simulink model "simTwoTag"  (R2023b)
settings: Solver=VariableStepAuto  StartTime=0.0  StopTime=10.0  RelTol=1e-3
undefined symbols (not defined in the file or in its folder): designMultirateFIR, get, hot, magnitude, paramWidebandRadar
libraries: phasedenvlib x4, phaseddetectlib x3, phasedtxrxlib x2, radarlib x2, simulink x1, phasedwavlib x1, dspobslib x1, dspmlti4 x1, dspsigops x1, dspmathops x1, phasedmisclib x1
settings Model: Creator=ericdvet  LastModifiedBy=ericdvet

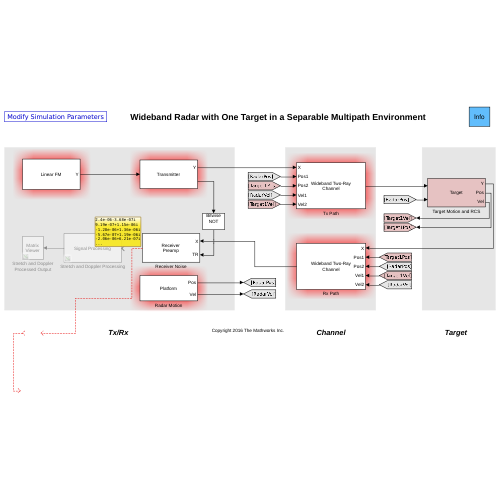
[thumbnail: Simulink's stored preview of the top-level diagram]
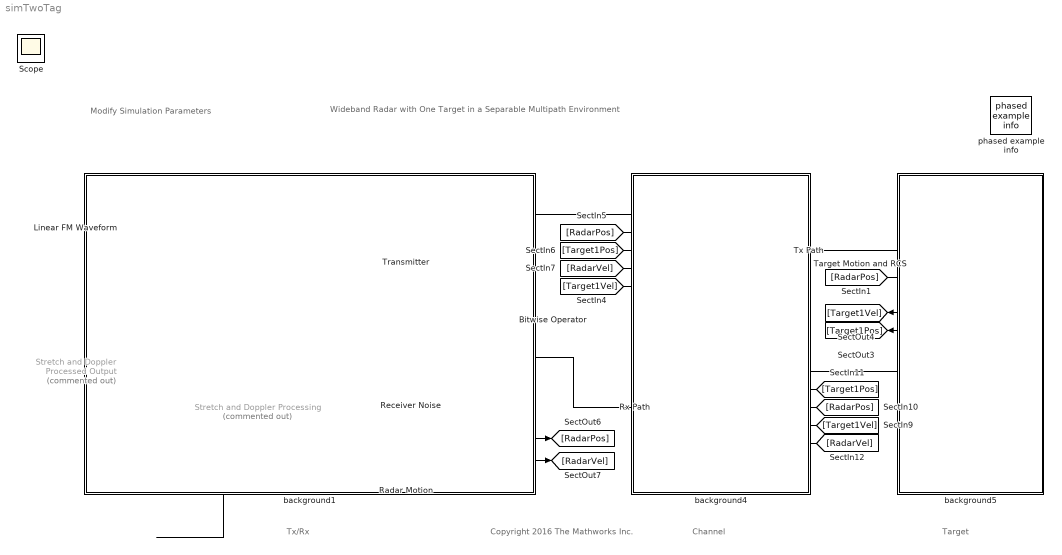
== system simTwoTag ==
  note: Wideband Radar with One Target in a Separable Multipath Environment
  note: Target
  note: Tx/Rx
  note: Copyright 2016 The Mathworks Inc.
  note: Modify Simulation Parameters
  note: Channel
  Bitwise Operator : simulink/Logic and Bit Operations/Bitwise Operator  logicop=NOT  UseBitMask=off  BitMask=bin2dec('11011001')  BitMaskRealWorld=Stored Integer
  Linear FM Waveform : phasedwavlib/Linear FM Waveform  SampleRate=paramWidebandRadar.fs  DurationSpecification=Pulse width  PulseWidth=paramWidebandRadar.pulseWidth  DutyCycle=0.5  PRF=paramWidebandRadar.prf  PRFSelectionInputPort=off  SimulationTimeSource=Derive from waveform parameters  SweepBandwidth=paramWidebandRadar.pulseBw  SweepDirection=Up  SweepInterval=Positive  Envelope=Rectangular  FrequencyOffsetSource=Property  FrequencyOffset=0  OutputFormat=Pulses  NumSamples=100  NumPulses=1  PRFOutputPort=off  CoefficientsOutputPort=off  SimulateUsing=Interpreted execution
  Radar Motion : phasedenvlib/Motion Platform  MotionModel=Velocity  InitialPosition=paramWidebandRadar.sensorPos  InitialVelocity=[ 0; 0; 0 ]  VelocitySource=Property  Velocity=paramWidebandRadar.sensorVel  AccelerationSource=Property  Acceleration=[0;0;0]  CustomTrajectory=[ 0, 0, 0, 0, 0, 0, 0; 1, 0, 0, 0, 0, 0, 0 ]  ScanMode=None  InitialScanAngle=0  AzimuthSpan=[ -60, 60 ]  AzimuthScanRate=10  InitialOrientationAxes=eye( 3 )  OrientationAxesOutputPort=off  ElapsedTimeSource=Auto  SampleRateFromInputCheckbox=on  SampleRate=1e6  SimulateUsing=Interpreted execution
  Receiver Noise : phasedtxrxlib/Receiver Preamp  Gain=20  LossFactor=0  NoiseMethod=Noise temperature  NoiseFigure=0  ReferenceTemperature=290  SampleRateFromInputCheckbox=on  SampleRate=1e6  NoisePower=0  EnableInputPort=on  PhaseNoiseInputPort=off  SeedSource=Auto  Seed=0  SimulateUsing=Interpreted execution
  Rx Path : radarlib/Wideband Two-Ray Channel  PropagationSpeed=paramWidebandRadar.propSpeed  OperatingFrequency=paramWidebandRadar.fc  NumSubbands=paramWidebandRadar.numSubbands  SpecifyAtmosphere=off  Temperature=15  DryAirPressure=101325  WaterVapourDensity=7.5  LiquidWaterDensity=0  RainRate=0  SampleRateFromInputCheckbox=on  SampleRate=1e6  GroundReflectionCoefficient=paramWidebandRadar.groundCoefficient  GroundRelativePermittivity=15  CombinedRaysOutput=on  MaximumDistanceSource=Property  MaximumDistance=10e3  MaximumNumInputSamplesSource=Auto  MaximumNumInputSamples=1000  SimulateUsing=Interpreted execution
  Stretch and Doppler Processed Output : dspobslib/Matrix Viewer  Commented=on  ImageParams=off  CMapStr=hot(256)  AxisColorbar=on  AxisParams=off  AxisOrigin=Lower left corner  AxisTickMode=User-defined  XTickRange=paramWidebandRadar.radialSpeedLim  YTickRange=paramWidebandRadar.rangeLim  XLabel=Radial Speed (m/s)  YLabel=Range (m)  ZLabel=SINR (dB)  FigPos=get(0,'defaultfigureposition')  AxisZoom=off
      settings: YMin=5  YMax=20
  Stretch and Doppler Processing : Subsystem  Commented=on
      mask Display: disp('Signal Processing')
  Target Motion and RCS : Subsystem
      mask Display:
      | disp('Target')
      | port_label('output',1,'Y');
      | port_label('output',2,'Pos');
      | port_label('output',3,'Vel');
  Transmitter : phasedtxrxlib/Transmitter  PeakPower=paramWidebandRadar.peakPower  Gain=paramWidebandRadar.txGain  LossFactor=0  InUseOutputPort=on  CoherentOnTransmit=on  PhaseNoiseOutputPort=off  SeedSource=Auto  Seed=0  SimulateUsing=Interpreted execution
  Tx Path : radarlib/Wideband Two-Ray Channel  PropagationSpeed=paramWidebandRadar.propSpeed  OperatingFrequency=paramWidebandRadar.fc  NumSubbands=paramWidebandRadar.numSubbands  SpecifyAtmosphere=off  Temperature=15  DryAirPressure=101325  WaterVapourDensity=7.5  LiquidWaterDensity=0  RainRate=0  SampleRateFromInputCheckbox=on  SampleRate=1e6  GroundReflectionCoefficient=paramWidebandRadar.groundCoefficient  GroundRelativePermittivity=15  CombinedRaysOutput=on  MaximumDistanceSource=Property  MaximumDistance=10e3  MaximumNumInputSamplesSource=Auto  MaximumNumInputSamples=1000  SimulateUsing=Interpreted execution
  background1 : Subsystem  Description=Jammer
      mask Display: disp('')
  background4 : Subsystem  Description=Jammer
      mask Display: disp('')
  background5 : Subsystem  Description=Jammer
      mask Display: disp('')
  phased example info : phasedmisclib/phased example info  SystemSampleTime=-1  VariantActivationTime=update diagram  AllowFlexibleInterface=on  Latency=0  AutoFrameSizeCalculation=off
  Scope : Scope
  wires:
  Bitwise Operator/1 -> Receiver Noise/2
  Radar Motion/2 -> [RadarVel]
  [Target1Pos] -> Tx Path/3
  Transmitter/2 -> Bitwise Operator/1
  Linear FM Waveform/1 -> Transmitter/1
  [Target1Pos] -> Rx Path/2
  Target Motion and RCS/2(Target Position) -> [Target1Pos]
  Target Motion and RCS/3(Target Velocity) -> [Target1Vel]
  [RadarPos] -> Tx Path/2
  Radar Motion/1 -> [RadarPos]
  Stretch and Doppler Processing/1(Out2) -> Stretch and Doppler Processed Output/1
  [RadarVel] -> Tx Path/4
  [RadarPos] -> Target Motion and RCS/2(In2)
  [Target1Vel] -> Tx Path/5
  [RadarPos] -> Rx Path/3
  Tx Path/1 -> Target Motion and RCS/1(In1)
  Target Motion and RCS/1(Out1) -> Rx Path/1
  [RadarVel] -> Rx Path/5
  [Target1Vel] -> Rx Path/4
  Transmitter/1 -> Tx Path/1
  Rx Path/1 -> Receiver Noise/1
  Receiver Noise/1 -> ?
  ? -> ?

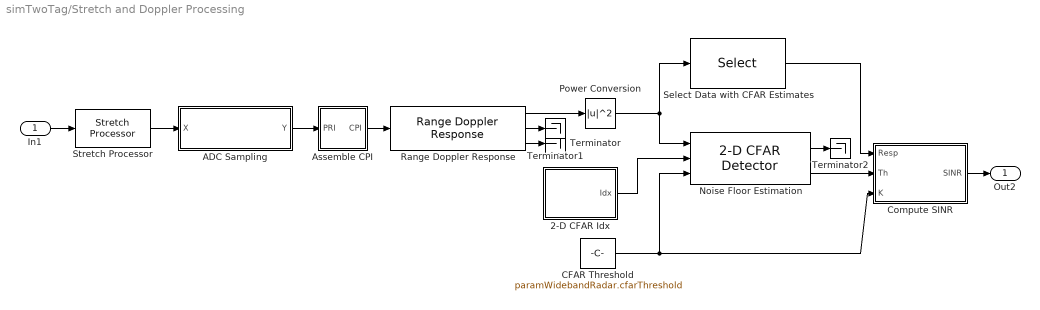
== system simTwoTag/Stretch and Doppler Processing ==
  In1 : Inport
  2-D CFAR Idx : MATLAB Function  TreatAsAtomicUnit=on  mask(2-D CFAR CUT Region){iCUTRng=paramWidebandRadar.cfarRngIdx(1):paramWidebandRadar.cfarRngIdx(2), iCUTDop=paramWidebandRadar.cfarSpdIdx(1):paramWidebandRadar.cfarSpdIdx(2)}
      mask prompts: iCUTRng "Range cells under test:"; iCUTDop "Doppler cells under test:"
      mask help: Generates 2-D CFAR CUT indicies to cover the 2-D region defined by the cell under test (CUT) indicies specified for both range and Doppler.
  ADC Sampling : Subsystem  mask(Decimator){M=paramWidebandRadar.decimateFactor}
      mask prompts: M "Decimation factor:"
      mask help: Decimates the sample rate of the received pulse repetition interval (PRI). The input is a column vector representing a full PRI. The output is a column vector representing the PRI sampled at a reduced rate. The reduction in the sampling rate is specified by the decimation factor, M.
      mask Display:
      | fprintf('Decimator');
      | port_label('input',1,'x[n]');
      | port_label('output',1,sprintf('x[%in]',M));
  Assemble CPI : Subsystem  mask(CPI Buffer){N=paramWidebandRadar.numPulseInt}
      mask prompts: N "PRIs per CPI"
      mask help: Buffers N pulse repetition intervals (PRIs) to form a coherent processing interval (CPI) to be used for Doppler processing. The input is a column vector representing a full PRI. The output is a 2-D column vector with each column corresponding to a buffered PRI.
      mask Display: fprintf('%i PRIs',N);
  CFAR Threshold : Constant  Value=paramWidebandRadar.cfarThreshold
  Compute SINR : Subsystem
  Noise Floor Estimation : phaseddetectlib/2-D CFAR Detector  Method=CA  Rank=paramWidebandRadar.cfarRank  GuardBandSize=paramWidebandRadar.numCFARGuard  TrainingBandSize=paramWidebandRadar.numCFARTrain  ThresholdFactor=Input port  ProbabilityFalseAlarm=0.1  CustomThresholdFactor=1  OutputFormat=CUT result  ThresholdOutputPort=on  NoisePowerOutputPort=off  NumDetectionsSource=Auto  NumDetections=1  SimulateUsing=Interpreted execution
  Power Conversion : Math  Operator=magnitude^2  SignedPower=on
  Range Doppler Response : phaseddetectlib/Range Doppler Response  RangeMethod=FFT  PropagationSpeed=paramWidebandRadar.propSpeed  SampleRateFromInputCheckbox=off  SampleRate=paramWidebandRadar.stretchFs  SweepSlope=paramWidebandRadar.stretchSlope  DechirpInput=off  RangeFFTLengthSource=Auto  RangeFFTLength=1024  RangeWindow=Taylor  RangeSidelobeAttenuation=30  CustomRangeWindow=@hamming  ReferenceRangeCentered=on  ReferenceRange=0  MaximumNumInputSamplesSource=Auto  MaximumNumInputSamples=100  PRFSource=Auto  PRF=10e3  DopplerFFTLengthSource=Property  DopplerFFTLength=paramWidebandRadar.numDopBins  DopplerWindow=Taylor  DopplerSidelobeAttenuation=30  CustomDopplerWindow=@hamming  DopplerOutput=Speed  OperatingFrequency=paramWidebandRadar.fc  SimulateUsing=Interpreted execution
  Select Data with CFAR Estimates : Selector  NumberOfDimensions=2  InputPortWidth=3  IndexOptions=Starting index (dialog),Starting index (dialog)  Indices=min(paramWidebandRadar.cfarRngIdx),min(paramWidebandRadar.cfarSpdIdx)  OutputSizes=max(paramWidebandRadar.cfarRngIdx)-min(paramWidebandRadar.cfarRngIdx)+1,max(paramWidebandRadar.cfarSpdIdx)-min(paramWidebandRadar.cfarSpdIdx)+1
  Stretch Processor : phaseddetectlib/Stretch Processor  PulseWidth=paramWidebandRadar.pulseWidth  PRFSource=Property  PRF=paramWidebandRadar.prf  SweepSlope=paramWidebandRadar.stretchSlope  SweepInterval=Positive  PropagationSpeed=paramWidebandRadar.propSpeed  ReferenceRange=paramWidebandRadar.stretchRef  RangeSpan=paramWidebandRadar.stretchSpan  SimulateUsing=Interpreted execution
  Terminator : Terminator
  Terminator1 : Terminator
  Terminator2 : Terminator
  Out2 : Outport
  wires:
  In1/1 -> Stretch Processor/1
  Assemble CPI/1(CPI) -> Range Doppler Response/1
  CFAR Threshold/1 -> Compute SINR/3(K), Noise Floor Estimation/3
  Noise Floor Estimation/1 -> Terminator2/1
  Range Doppler Response/3 -> Terminator/1
  Range Doppler Response/2 -> Terminator1/1
  Range Doppler Response/1 -> Power Conversion/1
  Select Data with CFAR Estimates/1 -> Compute SINR/1(Resp)
  Noise Floor Estimation/2 -> Compute SINR/2(Th)
  Compute SINR/1(SINR) -> Out2/1
  Power Conversion/1 -> Select Data with CFAR Estimates/1, Noise Floor Estimation/1
  Stretch Processor/1 -> ADC Sampling/1(X)
  ADC Sampling/1(Y) -> Assemble CPI/1(PRI)
  2-D CFAR Idx/1(Idx) -> Noise Floor Estimation/2

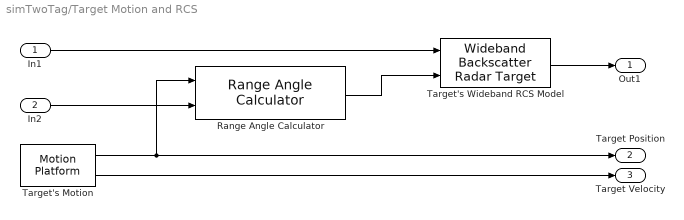
== system simTwoTag/Target Motion and RCS ==
  In1 : Inport
  In2 : Inport  Description=Radar Position  Port=2
  Range Angle Calculator : phasedenvlib/Range Angle Calculator  Model=Free space  ReferencePositionSource=Input port  ReferencePosition=[ 0; 0; 0 ]  ReferenceAxesSource=Property  ReferenceAxes=eye( 3 )  Output=Angle  SimulateUsing=Interpreted execution
  Target's Motion : phasedenvlib/Motion Platform  MotionModel=Velocity  InitialPosition=paramWidebandRadar.targetPos  InitialVelocity=[ 0; 0; 0 ]  VelocitySource=Property  Velocity=[0;0;0]  AccelerationSource=Property  Acceleration=[0;0;0]  CustomTrajectory=[ 0, 0, 0, 0, 0, 0, 0; 1, 0, 0, 0, 0, 0, 0 ]  ScanMode=None  InitialScanAngle=0  AzimuthSpan=[ -60, 60 ]  AzimuthScanRate=10  InitialOrientationAxes=eye( 3 )  OrientationAxesOutputPort=off  ElapsedTimeSource=Auto  SampleRateFromInputCheckbox=on  SampleRate=1e6  SimulateUsing=Interpreted execution
  Target's Wideband RCS Model : phasedenvlib/Wideband Backscatter Radar Target  EnablePolarization=off  FrequencyVector=paramWidebandRadar.rcsFreq  AzimuthAngles=paramWidebandRadar.rcsAz  ElevationAngles=paramWidebandRadar.rcsEl  RCSPattern=paramWidebandRadar.rcsPattern  ShhPattern=ones(181,361)  ShvPattern=ones(181,361)  SvvPattern=ones(181,361)  Model=Nonfluctuating  PropagationSpeed=paramWidebandRadar.propSpeed  OperatingFrequency=paramWidebandRadar.fc  SampleRateFromInputCheckbox=on  SampleRate=1e6  NumSubbands=paramWidebandRadar.numSubbands  SeedSource=Property  Seed=randi(65535,1)  SimulateUsing=Interpreted execution
  Out1 : Outport
  Target Position : Outport  Port=2
  Target Velocity : Outport  Port=3
  wires:
  Target's Motion/1 -> Range Angle Calculator/1, Target Position/1
  Target's Motion/2 -> Target Velocity/1
  In1/1 -> Target's Wideband RCS Model/1
  Target's Wideband RCS Model/1 -> Out1/1
  In2/1 -> Range Angle Calculator/2
  Range Angle Calculator/1 -> Target's Wideband RCS Model/2

== system simTwoTag/background1 ==

== system simTwoTag/background4 ==

== system simTwoTag/background5 ==

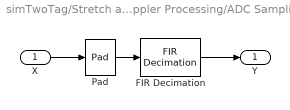
== system simTwoTag/Stretch and Doppler Processing/ADC Sampling ==
  X : Inport
  FIR Decimation : dspmlti4/FIR Decimation  FilterSource=Auto  h=designMultirateFIR(1,2)  D=M  filtStruct=Direct form  FilterObject=FDECIM  InputProcessing=Columns as channels (frame based)  framing=Enforce single-rate processing  AllowArbitraryInputLength=off  inputOffset=0  outputBufInitCond=0  roundingMode=Floor  overflowMode=off  firstCoeffDataTypeStr=Inherit: Same word length as input  firstCoeffMin=[]  firstCoeffMax=[]  firstCoeffLastDataTypeStr=Inherit: Same word length as input  outputDataTypeStr=Inherit: Same as accumulator  outputMin=[]  outputMax=[]  outputLastDataTypeStr=Inherit: Same as accumulator
  Pad : dspsigops/Pad  padAlong=Columns  dimsToPad=1  valSrc=Specify via dialog  padVal=0  spec=Output size  padNumOutRowsSpecMethod=User-specified  numOutRows=paramWidebandRadar.padLength  padNumOutColsSpecMethod=User-specified  numOutCols=paramWidebandRadar.priLength  isVarDimsMode=off  padBeginning=0  padEnd=0  outSizeMode=User-specified  outSize=1  padSigAt=End  trunc_flag=None  roundingMode=Floor  overflowMode=off  truncOrWrapMode=Truncate  wrap_flag=None
  Y : Outport
  wires:
  Pad/1 -> FIR Decimation/1
  FIR Decimation/1 -> Y/1
  X/1 -> Pad/1

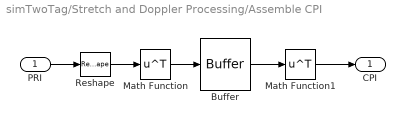
== system simTwoTag/Stretch and Doppler Processing/Assemble CPI ==
  PRI : Inport
  Buffer : Buffer  N=N
  Math Function : Math  Operator=transpose  SignedPower=on
  Math Function1 : Math  Operator=transpose  SignedPower=on
  Reshape : Reshape
  CPI : Outport
  wires:
  Math Function1/1 -> CPI/1
  Math Function/1 -> Buffer/1
  Reshape/1 -> Math Function/1
  Buffer/1 -> Math Function1/1
  PRI/1 -> Reshape/1

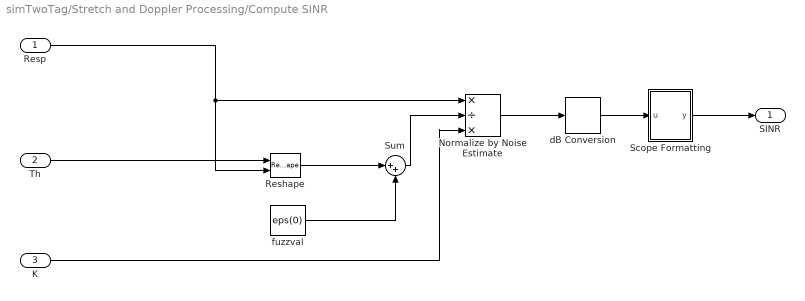
== system simTwoTag/Stretch and Doppler Processing/Compute SINR ==
  Resp : Inport
  Th : Inport  Port=2
  K : Inport  Port=3
  Normalize by Noise Estimate : Product  Inputs=*/*
  Reshape : Reshape  OutputDimensionality=Derive from reference input port
  Scope Formatting : MATLAB Function  TreatAsAtomicUnit=on
  Sum : Sum  Inputs=|++
  dB Conversion : dspmathops/dB Conversion  dBtype=dB  intype=Power  R=1  fuzz=on
  fuzzval : Constant  Value=eps(0)
  SINR : Outport
  wires:
  Resp/1 -> Reshape/2, Normalize by Noise Estimate/1
  K/1 -> Normalize by Noise Estimate/3
  Sum/1 -> Normalize by Noise Estimate/2
  fuzzval/1 -> Sum/2
  Th/1 -> Reshape/1
  Reshape/1 -> Sum/1
  dB Conversion/1 -> Scope Formatting/1(u)
  Scope Formatting/1(y) -> SINR/1
  Normalize by Noise Estimate/1 -> dB Conversion/1

== matlab function simTwoTag/Stretch and Doppler Processing/2-D CFAR Idx ==
  data: Idx output; iCUTRng parameter; iCUTDop parameter
function Idx = fcn(iCUTRng, iCUTDop)

% iCUTRng = 7923:8757;
% iCUTDop = 7:26;

% iCUTRng = cfarRngIdx(1):cfarRngIdx(2);
% iCUTDop = cfarSpdIdx(1):cfarSpdIdx(2);

[iRng, iDop] = meshgrid(iCUTRng,iCUTDop);
Idx = [iRng(:) iDop(:)]';

== matlab function simTwoTag/Stretch and Doppler Processing/Compute SINR/Scope Formatting ==
  data: u input; y output
function y = fcn(u)
%#codegen

y = rot90(u,2);
